simulink model "room2"  (R2021a)
settings: Solver=FixedStepAuto  StartTime=0.0  StopTime=10.0  RelTol=1e-3  EnableMultiTasking=on
libraries: dspmtrx3 x6, simulink x2
settings Model: DataDictionary=worldDD.sldd  SILPILModeSetting=veronly  ExtModeTrigDuration=2  Creator=Koorosh  LastModifiedBy=Koorosh
settings OptimizationCC: EnhancedBackFolding=on  PassReuseOutputArgsAs=Individual arguments  ZeroExternalMemoryAtStartup=off  ZeroInternalMemoryAtStartup=off  MaxStackSize=64  OptimizeBlockOrder=speed  DifferentSizesBufferReuse=on  OptimizationCustomize=off  EfficientTunableParamExpr=on
settings DebuggingCC: ParameterTunabilityLossMsg=error
settings HardwareCC: ProdBitPerInt=16  ProdBitPerPointer=16  ProdBitPerSizeT=16  ProdBitPerPtrDiffT=16  ProdLargestAtomicFloat=None  ProdWordSize=8  ProdHWDeviceType=Atmel->AVR
settings SFSimCC: MATLABDynamicMemAlloc=off
settings RTWCC: SystemTargetFile=ert.tlc  HardwareBoard=Arduino Uno  TemplateMakefile=ert_default_tmf  Toolchain=Arduino AVR  BuildConfiguration=Faster Runs
settings CodeAppCC: ForceParamTrailComments=on  IgnoreCustomStorageClasses=off  OperatorAnnotations=on  SimulinkDataObjDesc=on  SFDataObjDesc=on  InsertBlockDesc=on
settings ERTTargetCC: SupportContinuousTime=on  SupportVariableSizeSignals=on  ExtModeStaticAllocSize=250

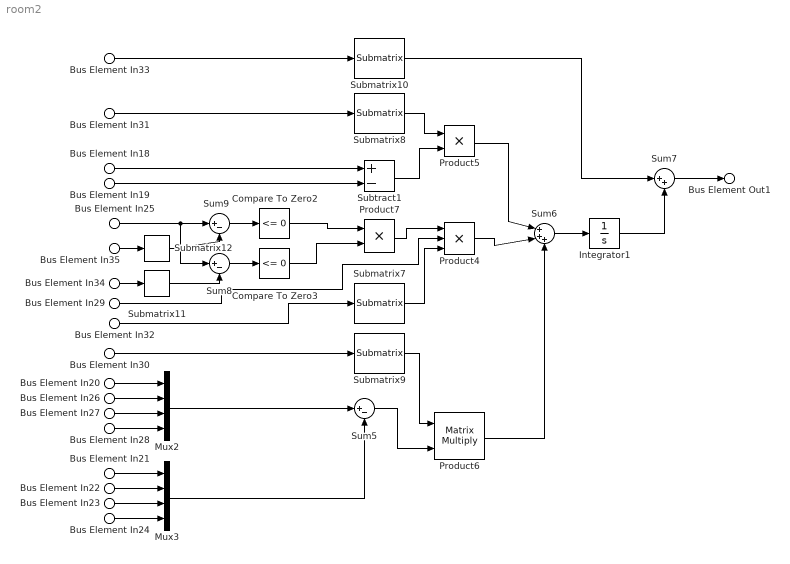
== system room2 ==
  Bus Element In18 : Inport  PortName=X  Element=u
  Bus Element In20 : Inport  PortName=X  Element=x1
  Bus Element In{19,21..26} (7 alike) : Inport  PortName=X  Element=x2
  Bus Element In27 : Inport  PortName=X  Element=x3
  Bus Element In28 : Inport  PortName=X  Element=x4
  Bus Element In29 : Inport  Port=2  PortName=H  Element=h2
  Bus Element In30 : Inport  Port=3  PortName=C  Element=A
  Bus Element In31 : Inport  Port=3  PortName=C  Element=b
  Bus Element In32 : Inport  Port=3  PortName=C  Element=c
  Bus Element In33 : Inport  Port=3  PortName=C  Element=x0
  Bus Element In34 : Inport  Port=3  PortName=C  Element=off
  Bus Element In35 : Inport  Port=3  PortName=C  Element=on
  Compare To Zero2 : simulink/Logic and Bit Operations/Compare To Zero  relop=<=  OutDataTypeStr=uint8
  Compare To Zero3 : simulink/Logic and Bit Operations/Compare To Zero  relop=<=  OutDataTypeStr=uint8
  Integrator1 : Integrator
  Mux2 : Mux
  Mux3 : Mux
  Product4 : Product  Inputs=3
  Product5 : Product
  Product6 : Product  Multiplication=Matrix(*)
  Product7 : Product
  Submatrix{7..8,10..12} (5 alike) : dspmtrx3/Submatrix  RowSpan=One row  RowStartMode=Index  RowStartIndex=2  RowEndMode=Last  RowEndIndex=1  ColSpan=One column  ColStartMode=First  ColStartIndex=1  ColEndMode=Last  ColEndIndex=1
  Submatrix9 : dspmtrx3/Submatrix  RowSpan=One row  RowStartMode=Index  RowStartIndex=2  RowEndMode=Last  RowEndIndex=1  ColSpan=All columns  ColStartMode=First  ColStartIndex=1  ColEndMode=Last  ColEndIndex=1
  Subtract1 : Sum  Inputs=+-
  Sum5 : Sum  Inputs=|+-
  Sum6 : Sum  Inputs=|+++
  Sum7 : Sum  Inputs=|++
  Sum8 : Sum  Inputs=|+-
  Sum9 : Sum  Inputs=|+-
  Bus Element Out1 : Outport  PortName=x2
  wires:
  Bus Element In29/1 -> Product4/2
  Submatrix12/1 -> Sum9/2
  Product7/1 -> Product4/1
  Bus Element In26/1 -> Mux2/2
  Bus Element In35/1 -> Submatrix12/1
  Submatrix10/1 -> Sum7/1
  Bus Element In21/1 -> Mux3/1
  Sum5/1 -> Product6/2
  Integrator1/1 -> Sum7/2
  Sum9/1 -> Compare To Zero2/1
  Bus Element In27/1 -> Mux2/3
  Submatrix7/1 -> Product4/3
  Submatrix11/1 -> Sum8/2
  Mux3/1 -> Sum5/2
  Product6/1 -> Sum6/3
  Bus Element In33/1 -> Submatrix10/1
  Sum8/1 -> Compare To Zero3/1
  Sum6/1 -> Integrator1/1
  Bus Element In22/1 -> Mux3/2
  Submatrix8/1 -> Product5/1
  Subtract1/1 -> Product5/2
  Bus Element In20/1 -> Mux2/1
  Bus Element In19/1 -> Subtract1/2
  Product4/1 -> Sum6/2
  Bus Element In34/1 -> Submatrix11/1
  Bus Element In18/1 -> Subtract1/1
  Bus Element In28/1 -> Mux2/4
  Submatrix9/1 -> Product6/1
  Bus Element In23/1 -> Mux3/3
  Bus Element In24/1 -> Mux3/4
  Mux2/1 -> Sum5/1
  Bus Element In25/1 -> Sum8/1, Sum9/1
  Bus Element In31/1 -> Submatrix8/1
  Bus Element In32/1 -> Submatrix7/1
  Product5/1 -> Sum6/1
  Bus Element In30/1 -> Submatrix9/1
  Sum7/1 -> Bus Element Out1/1
  Compare To Zero2/1 -> Product7/1
  Compare To Zero3/1 -> Product7/2
